simulink model "SlidingMode_Sim"  (R2018a)
settings: Solver=ode45  StartTime=0.0  StopTime=20  MaxStep=1e-4  RelTol=1e-3  EnableMultiTasking=on
values from neighbouring files (symbols this model uses):
  alpha = (3*Pa)/(4*a*Pb)    (= 3.41538461538)    [variables.m]
  epsi = 0.001    [variables.m]
  g = 9.81    [variables.m]
  Pa = 1.184    [variables.m]
  Pb = 10.4    [variables.m]
settings Model: Creator=Gabriel  LastModifiedBy=mpfva
settings SolverCC: ZeroCrossControl=DisableAll
settings DataIOCC: LimitDataPoints=on  SaveFormat=Array
settings OptimizationCC: LifeSpan=inf
settings DebuggingCC: UnderspecifiedInitializationDetection=Classic  MergeDetectMultiDrivingBlocksExec=none  SolverPrmCheckMsg=warning  StateNameClashWarn=warning  SFUnexpectedBacktrackingDiag=warning  SFNoUnconditionalDefaultTransitionDiag=warning  SFExecutionAtInitializationDiag=none
settings HardwareCC: ProdBitPerPointer=32  ProdBitPerSizeT=32  ProdBitPerPtrDiffT=32  ProdLargestAtomicFloat=None  ProdIntDivRoundTo=Undefined  ProdEndianess=Unspecified  ProdWordSize=32  ProdHWDeviceType=32-bit Generic
settings ModelReferenceCC: PropagateSignalLabelsOutOfModel=off
settings CodeAppCC: StateflowObjectComments=on
settings GRTTargetCC: TargetLangStandard=C89/C90 (ANSI)  GeneratePreprocessorConditionals=Disable all
settings ConfigComp: CovMetricSettings=dw  CovHtmlReporting=on  CovSaveCumulativeToWorkspaceVar=on  CovSaveSingleToWorkspaceVar=on  CovExternalEMLEnable=off

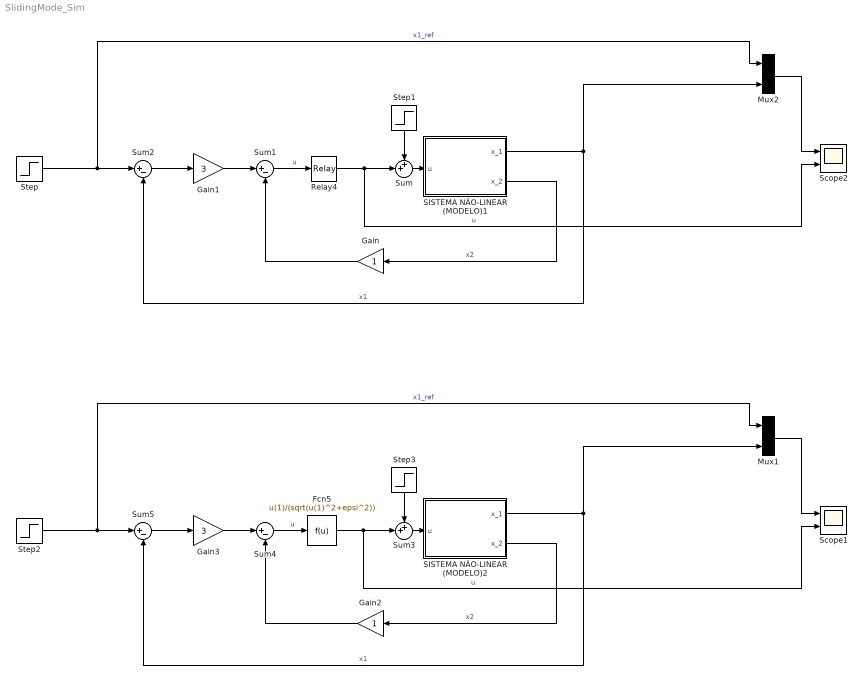
== system SlidingMode_Sim ==
  Fcn5 : Fcn  Expr=u(1)/(sqrt(u(1)^2+epsi^2))
  Gain : Gain
  Gain1 : Gain  Gain=3
  Gain2 : Gain
  Gain3 : Gain  Gain=3
  Mux1 : Mux  Inputs=2
  Mux2 : Mux  Inputs=2
  Relay4 : Relay  OnSwitchValue=0.1  OffSwitchValue=-0.1  OffOutputValue=-1
  SISTEMA NÃO-LINEAR (MODELO)1 : Subsystem
  SISTEMA NÃO-LINEAR (MODELO)2 : Subsystem
  Scope1 : Scope  NumInputPorts=2
  Scope2 : Scope  NumInputPorts=2
  Step : Step  Time=0  After=0.6  SampleTime=0
  Step1 : Step  Time=0  SampleTime=0
  Step2 : Step  Time=0  After=0.6  SampleTime=0
  Step3 : Step  Time=0  SampleTime=0
  Sum : Sum  Inputs=++|
  Sum{1..2,4..5} (4 alike) : Sum  Inputs=|+-
  Sum3 : Sum  Inputs=++|
  wires:
  Sum1/1 -> Relay4/1  "u"
  Step/1 -> Mux2/1, Sum2/1  "x1_ref"
  Mux2/1 -> Scope2/1
  SISTEMA NÃO-LINEAR (MODELO)1/1(x_1) -> Sum2/2, Mux2/2  "x1"
  SISTEMA NÃO-LINEAR (MODELO)1/2(x_2) -> Gain/1  "x2"
  Gain1/1 -> Sum1/1
  Gain/1 -> Sum1/2
  Sum2/1 -> Gain1/1
  Sum/1 -> SISTEMA NÃO-LINEAR (MODELO)1/1(u)
  Step1/1 -> Sum/1
  Relay4/1 -> Scope2/2, Sum/2  "u"
  Sum4/1 -> Fcn5/1  "u"
  Sum3/1 -> SISTEMA NÃO-LINEAR (MODELO)2/1(u)
  Sum5/1 -> Gain3/1
  SISTEMA NÃO-LINEAR (MODELO)2/2(x_2) -> Gain2/1  "x2"
  Fcn5/1 -> Scope1/2, Sum3/2  "u"
  SISTEMA NÃO-LINEAR (MODELO)2/1(x_1) -> Sum5/2, Mux1/2  "x1"
  Gain2/1 -> Sum4/2
  Gain3/1 -> Sum4/1
  Mux1/1 -> Scope1/1
  Step3/1 -> Sum3/1
  Step2/1 -> Mux1/1, Sum5/1  "x1_ref"

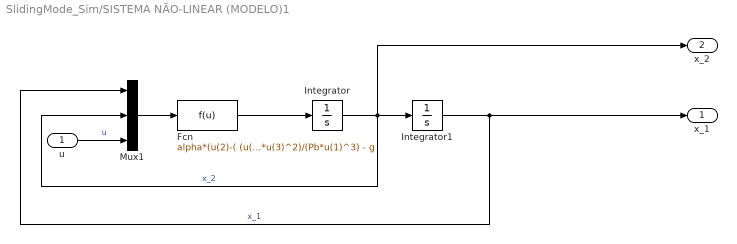
== system SlidingMode_Sim/SISTEMA NÃO-LINEAR (MODELO)1 ==
  u : Inport
  Fcn : Fcn  Expr=alpha*(u(2)-( (u(3))/u(1)) )^2 - (Pa*u(3)^2)/(Pb*u(1)^3) - g
  Integrator : Integrator
  Integrator1 : Integrator  InitialCondition=0.1  LimitOutput=on  UpperSaturationLimit=2  LowerSaturationLimit=0.001
  Mux1 : Mux  Inputs=3
  x_1 : Outport
  x_2 : Outport  Port=2
  wires:
  Fcn/1 -> Integrator/1
  Integrator/1 -> Mux1/2, x_2/1, Integrator1/1  "x_2"
  u/1 -> Mux1/3  "u"
  Mux1/1 -> Fcn/1
  Integrator1/1 -> Mux1/1, x_1/1  "x_1"

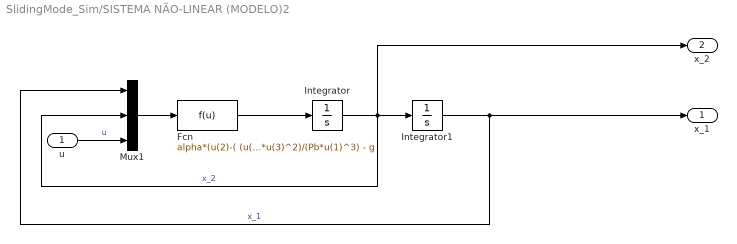
== system SlidingMode_Sim/SISTEMA NÃO-LINEAR (MODELO)2 ==
  u : Inport
  Fcn : Fcn  Expr=alpha*(u(2)-( (u(3))/u(1)) )^2 - (Pa*u(3)^2)/(Pb*u(1)^3) - g
  Integrator : Integrator
  Integrator1 : Integrator  InitialCondition=0.1  LimitOutput=on  UpperSaturationLimit=2  LowerSaturationLimit=0.001
  Mux1 : Mux  Inputs=3
  x_1 : Outport
  x_2 : Outport  Port=2
  wires:
  Fcn/1 -> Integrator/1
  Integrator/1 -> Mux1/2, x_2/1, Integrator1/1  "x_2"
  u/1 -> Mux1/3  "u"
  Mux1/1 -> Fcn/1
  Integrator1/1 -> Mux1/1, x_1/1  "x_1"
